simulink model "database_init"  (R2023a)
settings: configuration reference "config" (kept outside this file)
model workspace (MAT data in the model file):
  timer_s = Simulink.Signal
  timer_s.Description = '时间计数器 s'
  timer_s.DataType = 'single'
  timer_s.Dimensions = -1
  timer_s.DimensionsMode = 'auto'
  timer_s.Complexity = 'auto'
  timer_s.SampleTime = -1
  timer_s.SamplingMode = 'auto'
  timer_s.InitialValue = '0'
settings Model: DataDictionary=model_config.sldd  Creator=huangcheng  LastModifiedBy=Administrator
settings ConfigSetRef: SourceName=config

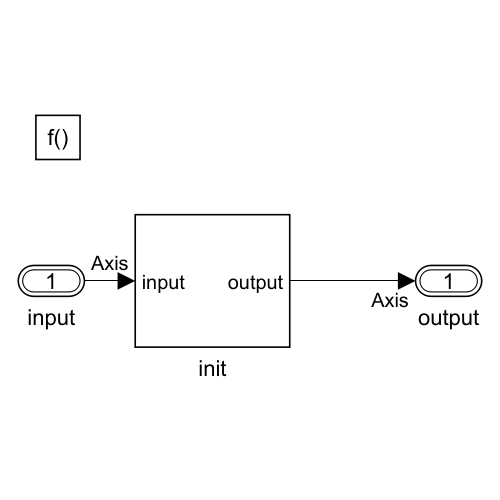
[thumbnail: Simulink's stored preview of the top-level diagram]
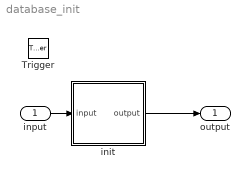
== system database_init ==
  input : Inport  OutDataTypeStr=Bus: Axis  BusOutputAsStruct=on
  Trigger : TriggerPort  TriggerType=function-call  VariantControl=(inherit)  PortDimensions=1
  init : Subsystem
  output : Outport  OutDataTypeStr=Bus: Axis  BusOutputAsStruct=on
  wires:
  input/1 -> init/1(input)
  init/1(output) -> output/1

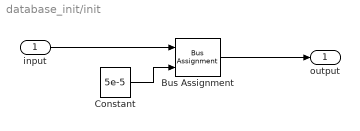
== system database_init/init ==
  input : Inport
  Bus Assignment : BusAssignment  AssignedSignals=current_ctl_config.dt_s
  Constant : Constant  Value=5e-5  OutDataTypeStr=single  SampleTime=-1
  output : Outport
  wires:
  Constant/1 -> Bus Assignment/2
  Bus Assignment/1 -> output/1
  input/1 -> Bus Assignment/1
